simulink model "Karatsuba_Multiplier_64_Unsigned"  (R2012b)
settings: Solver=FixedStepDiscrete  SolverMode=SingleTasking  StartTime=0  StopTime=stopClock  RelTol=1e-3
libraries: xbsIndex_r4 x469
(part 2 of 3)

== system Karatsuba_Multiplier_64_Unsigned/AE_Multiplier_32_0/Barrel Shifter 9 ==
  Sel : Inport
  x : Inport  Port=2
  Mux : xbsIndex_r4/Mux  inputs=8  en=off  latency=0  precision=Full  arith_type=Unsigned  n_bits=17  bin_pt=0  quantization=Truncate  overflow=Wrap  dbl_ovrd=off  block_type=mux
  Shift1 : xbsIndex_r4/Shift  shift_dir=Left  shift_bits=1  en=off  latency=0  precision=User Defined  arith_type=Unsigned  n_bits=64  bin_pt=0  quantization=Truncate  overflow=Wrap  dbl_ovrd=off  block_type=shift
  Shift2 : xbsIndex_r4/Shift  shift_dir=Left  shift_bits=2  en=off  latency=0  precision=User Defined  arith_type=Unsigned  n_bits=64  bin_pt=0  quantization=Truncate  overflow=Wrap  dbl_ovrd=off  block_type=shift
  Shift3 : xbsIndex_r4/Shift  shift_dir=Left  shift_bits=3  en=off  latency=0  precision=User Defined  arith_type="Signed  (2's comp)"  n_bits=64  bin_pt=0  quantization=Truncate  overflow=Wrap  dbl_ovrd=off  block_type=shift
  Shift4 : xbsIndex_r4/Shift  shift_dir=Left  shift_bits=4  en=off  latency=0  precision=User Defined  arith_type=Unsigned  n_bits=64  bin_pt=0  quantization=Truncate  overflow=Wrap  dbl_ovrd=off  block_type=shift
  Shift5 : xbsIndex_r4/Shift  shift_dir=Left  shift_bits=5  en=off  latency=0  precision=User Defined  arith_type=Unsigned  n_bits=43  bin_pt=0  quantization=Truncate  overflow=Wrap  dbl_ovrd=off  block_type=shift
  Shift6 : xbsIndex_r4/Shift  shift_dir=Left  shift_bits=6  en=off  latency=0  precision=User Defined  arith_type=Unsigned  n_bits=64  bin_pt=0  quantization=Truncate  overflow=Wrap  dbl_ovrd=off  block_type=shift
  Shift7 : xbsIndex_r4/Shift  shift_dir=Left  shift_bits=7  en=off  latency=0  precision=User Defined  arith_type=Unsigned  n_bits=64  bin_pt=0  quantization=Truncate  overflow=Wrap  dbl_ovrd=off  block_type=shift
  y : Outport
  wires:
  Mux/1 -> y/1
  Sel/1 -> Mux/1
  x/1 -> Shift1/1, Shift2/1, Shift3/1, Shift4/1, Shift5/1, Shift6/1, Shift7/1, Mux/2
  Shift1/1 -> Mux/3
  Shift2/1 -> Mux/4
  Shift3/1 -> Mux/5
  Shift4/1 -> Mux/6
  Shift5/1 -> Mux/7
  Shift6/1 -> Mux/8
  Shift7/1 -> Mux/9

== system Karatsuba_Multiplier_64_Unsigned/AE_Multiplier_32_0/Encoder Slicer0 ==
  x : Inport
  Slice Enc a1 : xbsIndex_r4/Slice  nbits=3  boolean_output=off  mode=Lower Bit Location + Width  bit1=0  base1=MSB of Input  bit0=6  base0=LSB of Input  dbl_ovrd=off  block_type=slice
  Slice Enc a2 : xbsIndex_r4/Slice  nbits=3  boolean_output=off  mode=Lower Bit Location + Width  bit1=0  base1=MSB of Input  bit0=0  base0=LSB of Input  dbl_ovrd=off  block_type=slice
  Slice Enc s2 : xbsIndex_r4/Slice  nbits=1  boolean_output=on  mode=Lower Bit Location + Width  bit1=0  base1=MSB of Input  bit0=3  base0=LSB of Input  dbl_ovrd=off  block_type=slice
  Slice Enc t1 : xbsIndex_r4/Slice  nbits=2  boolean_output=off  mode=Upper Bit Location + Width  bit1=0  base1=MSB of Input  bit0=0  base0=MSB of Input  dbl_ovrd=off  block_type=slice
  Slice Enc t2 : xbsIndex_r4/Slice  nbits=2  boolean_output=off  mode=Lower Bit Location + Width  bit1=0  base1=MSB of Input  bit0=4  base0=LSB of Input  dbl_ovrd=off  block_type=slice
  t1 : Outport
  a1 : Outport  Port=2
  t2 : Outport  Port=3
  a2 : Outport  Port=4
  s2 : Outport  Port=5
  wires:
  Slice Enc t2/1 -> t2/1
  Slice Enc a1/1 -> a1/1
  Slice Enc a2/1 -> a2/1
  Slice Enc t1/1 -> t1/1
  Slice Enc s2/1 -> s2/1
  x/1 -> Slice Enc s2/1, Slice Enc a2/1, Slice Enc t1/1, Slice Enc a1/1, Slice Enc t2/1

== system Karatsuba_Multiplier_64_Unsigned/AE_Multiplier_32_0/Encoder Slicer1 ==
  x : Inport
  Slice Enc a1 : xbsIndex_r4/Slice  nbits=3  boolean_output=off  mode=Lower Bit Location + Width  bit1=0  base1=MSB of Input  bit0=6  base0=LSB of Input  dbl_ovrd=off  block_type=slice
  Slice Enc a2 : xbsIndex_r4/Slice  nbits=3  boolean_output=off  mode=Lower Bit Location + Width  bit1=0  base1=MSB of Input  bit0=0  base0=LSB of Input  dbl_ovrd=off  block_type=slice
  Slice Enc s2 : xbsIndex_r4/Slice  nbits=1  boolean_output=on  mode=Lower Bit Location + Width  bit1=0  base1=MSB of Input  bit0=3  base0=LSB of Input  dbl_ovrd=off  block_type=slice
  Slice Enc t1 : xbsIndex_r4/Slice  nbits=2  boolean_output=off  mode=Upper Bit Location + Width  bit1=0  base1=MSB of Input  bit0=0  base0=MSB of Input  dbl_ovrd=off  block_type=slice
  Slice Enc t2 : xbsIndex_r4/Slice  nbits=2  boolean_output=off  mode=Lower Bit Location + Width  bit1=0  base1=MSB of Input  bit0=4  base0=LSB of Input  dbl_ovrd=off  block_type=slice
  t1 : Outport
  a1 : Outport  Port=2
  t2 : Outport  Port=3
  a2 : Outport  Port=4
  s2 : Outport  Port=5
  wires:
  Slice Enc t2/1 -> t2/1
  Slice Enc a1/1 -> a1/1
  Slice Enc a2/1 -> a2/1
  Slice Enc t1/1 -> t1/1
  Slice Enc s2/1 -> s2/1
  x/1 -> Slice Enc s2/1, Slice Enc a2/1, Slice Enc t1/1, Slice Enc a1/1, Slice Enc t2/1

== system Karatsuba_Multiplier_64_Unsigned/AE_Multiplier_32_0/Encoder Slicer2 ==
  x : Inport
  Slice Enc a1 : xbsIndex_r4/Slice  nbits=3  boolean_output=off  mode=Lower Bit Location + Width  bit1=0  base1=MSB of Input  bit0=6  base0=LSB of Input  dbl_ovrd=off  block_type=slice
  Slice Enc a2 : xbsIndex_r4/Slice  nbits=3  boolean_output=off  mode=Lower Bit Location + Width  bit1=0  base1=MSB of Input  bit0=0  base0=LSB of Input  dbl_ovrd=off  block_type=slice
  Slice Enc s2 : xbsIndex_r4/Slice  nbits=1  boolean_output=on  mode=Lower Bit Location + Width  bit1=0  base1=MSB of Input  bit0=3  base0=LSB of Input  dbl_ovrd=off  block_type=slice
  Slice Enc t1 : xbsIndex_r4/Slice  nbits=2  boolean_output=off  mode=Upper Bit Location + Width  bit1=0  base1=MSB of Input  bit0=0  base0=MSB of Input  dbl_ovrd=off  block_type=slice
  Slice Enc t2 : xbsIndex_r4/Slice  nbits=2  boolean_output=off  mode=Lower Bit Location + Width  bit1=0  base1=MSB of Input  bit0=4  base0=LSB of Input  dbl_ovrd=off  block_type=slice
  t1 : Outport
  a1 : Outport  Port=2
  t2 : Outport  Port=3
  a2 : Outport  Port=4
  s2 : Outport  Port=5
  wires:
  Slice Enc t2/1 -> t2/1
  Slice Enc a1/1 -> a1/1
  Slice Enc a2/1 -> a2/1
  Slice Enc t1/1 -> t1/1
  Slice Enc s2/1 -> s2/1
  x/1 -> Slice Enc s2/1, Slice Enc a2/1, Slice Enc t1/1, Slice Enc a1/1, Slice Enc t2/1

== system Karatsuba_Multiplier_64_Unsigned/AE_Multiplier_32_0/Encoder Slicer3 ==
  x : Inport
  Slice Enc a1 : xbsIndex_r4/Slice  nbits=3  boolean_output=off  mode=Lower Bit Location + Width  bit1=0  base1=MSB of Input  bit0=6  base0=LSB of Input  dbl_ovrd=off  block_type=slice
  Slice Enc a2 : xbsIndex_r4/Slice  nbits=3  boolean_output=off  mode=Lower Bit Location + Width  bit1=0  base1=MSB of Input  bit0=0  base0=LSB of Input  dbl_ovrd=off  block_type=slice
  Slice Enc s2 : xbsIndex_r4/Slice  nbits=1  boolean_output=on  mode=Lower Bit Location + Width  bit1=0  base1=MSB of Input  bit0=3  base0=LSB of Input  dbl_ovrd=off  block_type=slice
  Slice Enc t1 : xbsIndex_r4/Slice  nbits=2  boolean_output=off  mode=Upper Bit Location + Width  bit1=0  base1=MSB of Input  bit0=0  base0=MSB of Input  dbl_ovrd=off  block_type=slice
  Slice Enc t2 : xbsIndex_r4/Slice  nbits=2  boolean_output=off  mode=Lower Bit Location + Width  bit1=0  base1=MSB of Input  bit0=4  base0=LSB of Input  dbl_ovrd=off  block_type=slice
  t1 : Outport
  a1 : Outport  Port=2
  t2 : Outport  Port=3
  a2 : Outport  Port=4
  s2 : Outport  Port=5
  wires:
  Slice Enc t2/1 -> t2/1
  Slice Enc a1/1 -> a1/1
  Slice Enc a2/1 -> a2/1
  Slice Enc t1/1 -> t1/1
  Slice Enc s2/1 -> s2/1
  x/1 -> Slice Enc s2/1, Slice Enc a2/1, Slice Enc t1/1, Slice Enc a1/1, Slice Enc t2/1

== system Karatsuba_Multiplier_64_Unsigned/AE_Multiplier_32_0/Encoder Slicer4 ==
  x : Inport
  Slice Enc a1 : xbsIndex_r4/Slice  nbits=3  boolean_output=off  mode=Lower Bit Location + Width  bit1=0  base1=MSB of Input  bit0=6  base0=LSB of Input  dbl_ovrd=off  block_type=slice
  Slice Enc a2 : xbsIndex_r4/Slice  nbits=3  boolean_output=off  mode=Lower Bit Location + Width  bit1=0  base1=MSB of Input  bit0=0  base0=LSB of Input  dbl_ovrd=off  block_type=slice
  Slice Enc s2 : xbsIndex_r4/Slice  nbits=1  boolean_output=on  mode=Lower Bit Location + Width  bit1=0  base1=MSB of Input  bit0=3  base0=LSB of Input  dbl_ovrd=off  block_type=slice
  Slice Enc t1 : xbsIndex_r4/Slice  nbits=2  boolean_output=off  mode=Upper Bit Location + Width  bit1=0  base1=MSB of Input  bit0=0  base0=MSB of Input  dbl_ovrd=off  block_type=slice
  Slice Enc t2 : xbsIndex_r4/Slice  nbits=2  boolean_output=off  mode=Lower Bit Location + Width  bit1=0  base1=MSB of Input  bit0=4  base0=LSB of Input  dbl_ovrd=off  block_type=slice
  t1 : Outport
  a1 : Outport  Port=2
  t2 : Outport  Port=3
  a2 : Outport  Port=4
  s2 : Outport  Port=5
  wires:
  Slice Enc t2/1 -> t2/1
  Slice Enc a1/1 -> a1/1
  Slice Enc a2/1 -> a2/1
  Slice Enc t1/1 -> t1/1
  Slice Enc s2/1 -> s2/1
  x/1 -> Slice Enc s2/1, Slice Enc a2/1, Slice Enc t1/1, Slice Enc a1/1, Slice Enc t2/1

== system Karatsuba_Multiplier_64_Unsigned/AE_Multiplier_32_1/3B Multiplier ==
  x : Inport
  AddSub : xbsIndex_r4/AddSub  mode=Addition  use_carryin=off  use_carryout=off  en=off  latency=0  precision=User Defined  arith_type=Unsigned  n_bits=64  bin_pt=0  quantization=Truncate  overflow=Wrap  dbl_ovrd=off  use_behavioral_HDL=off  hw_selection=Fabric  pipelined=on  block_type=addsub
  Shift : xbsIndex_r4/Shift  shift_dir=Left  shift_bits=1  en=off  latency=0  precision=User Defined  arith_type=Unsigned  n_bits=64  bin_pt=0  quantization=Truncate  overflow=Wrap  dbl_ovrd=off  block_type=shift
  y : Outport
  wires:
  x/1 -> Shift/1, AddSub/2
  AddSub/1 -> y/1
  Shift/1 -> AddSub/1

== system Karatsuba_Multiplier_64_Unsigned/AE_Multiplier_32_1/5B Multiplier ==
  x : Inport
  AddSub1 : xbsIndex_r4/AddSub  mode=Addition  use_carryin=off  use_carryout=off  en=off  latency=0  precision=User Defined  arith_type=Unsigned  n_bits=64  bin_pt=0  quantization=Truncate  overflow=Wrap  dbl_ovrd=off  use_behavioral_HDL=off  hw_selection=Fabric  pipelined=on  block_type=addsub
  Shift1 : xbsIndex_r4/Shift  shift_dir=Left  shift_bits=2  en=off  latency=0  precision=User Defined  arith_type=Unsigned  n_bits=64  bin_pt=0  quantization=Truncate  overflow=Wrap  dbl_ovrd=off  block_type=shift
  y : Outport
  wires:
  x/1 -> AddSub1/2, Shift1/1
  Shift1/1 -> AddSub1/1
  AddSub1/1 -> y/1

== system Karatsuba_Multiplier_64_Unsigned/AE_Multiplier_32_1/7B Multiplier ==
  x : Inport
  AddSub2 : xbsIndex_r4/AddSub  mode=Subtraction  use_carryin=off  use_carryout=off  en=off  latency=0  precision=User Defined  arith_type=Unsigned  n_bits=64  bin_pt=0  quantization=Truncate  overflow=Wrap  dbl_ovrd=off  use_behavioral_HDL=off  hw_selection=Fabric  pipelined=on  block_type=addsub
  Shift2 : xbsIndex_r4/Shift  shift_dir=Left  shift_bits=3  en=off  latency=0  precision=User Defined  arith_type=Unsigned  n_bits=64  bin_pt=0  quantization=Truncate  overflow=Wrap  dbl_ovrd=off  block_type=shift
  y : Outport
  wires:
  AddSub2/1 -> y/1
  Shift2/1 -> AddSub2/1
  x/1 -> Shift2/1, AddSub2/2

== system Karatsuba_Multiplier_64_Unsigned/AE_Multiplier_32_1/Barrel Shifter 0 ==
  Sel : Inport
  x : Inport  Port=2
  Mux : xbsIndex_r4/Mux  inputs=8  en=off  latency=0  precision=Full  arith_type=Unsigned  n_bits=17  bin_pt=0  quantization=Truncate  overflow=Wrap  dbl_ovrd=off  block_type=mux
  Shift1 : xbsIndex_r4/Shift  shift_dir=Left  shift_bits=1  en=off  latency=0  precision=User Defined  arith_type=Unsigned  n_bits=64  bin_pt=0  quantization=Truncate  overflow=Wrap  dbl_ovrd=off  block_type=shift
  Shift2 : xbsIndex_r4/Shift  shift_dir=Left  shift_bits=2  en=off  latency=0  precision=User Defined  arith_type=Unsigned  n_bits=64  bin_pt=0  quantization=Truncate  overflow=Wrap  dbl_ovrd=off  block_type=shift
  Shift3 : xbsIndex_r4/Shift  shift_dir=Left  shift_bits=3  en=off  latency=0  precision=User Defined  arith_type="Signed  (2's comp)"  n_bits=64  bin_pt=0  quantization=Truncate  overflow=Wrap  dbl_ovrd=off  block_type=shift
  Shift4 : xbsIndex_r4/Shift  shift_dir=Left  shift_bits=4  en=off  latency=0  precision=User Defined  arith_type=Unsigned  n_bits=64  bin_pt=0  quantization=Truncate  overflow=Wrap  dbl_ovrd=off  block_type=shift
  Shift5 : xbsIndex_r4/Shift  shift_dir=Left  shift_bits=5  en=off  latency=0  precision=User Defined  arith_type=Unsigned  n_bits=43  bin_pt=0  quantization=Truncate  overflow=Wrap  dbl_ovrd=off  block_type=shift
  Shift6 : xbsIndex_r4/Shift  shift_dir=Left  shift_bits=6  en=off  latency=0  precision=User Defined  arith_type=Unsigned  n_bits=64  bin_pt=0  quantization=Truncate  overflow=Wrap  dbl_ovrd=off  block_type=shift
  Shift7 : xbsIndex_r4/Shift  shift_dir=Left  shift_bits=7  en=off  latency=0  precision=User Defined  arith_type=Unsigned  n_bits=64  bin_pt=0  quantization=Truncate  overflow=Wrap  dbl_ovrd=off  block_type=shift
  y : Outport
  wires:
  Mux/1 -> y/1
  Sel/1 -> Mux/1
  x/1 -> Shift1/1, Shift2/1, Shift3/1, Shift4/1, Shift5/1, Shift6/1, Shift7/1, Mux/2
  Shift1/1 -> Mux/3
  Shift2/1 -> Mux/4
  Shift3/1 -> Mux/5
  Shift4/1 -> Mux/6
  Shift5/1 -> Mux/7
  Shift6/1 -> Mux/8
  Shift7/1 -> Mux/9

== system Karatsuba_Multiplier_64_Unsigned/AE_Multiplier_32_1/Barrel Shifter 1 ==
  Sel : Inport
  x : Inport  Port=2
  Mux : xbsIndex_r4/Mux  inputs=8  en=off  latency=0  precision=Full  arith_type=Unsigned  n_bits=17  bin_pt=0  quantization=Truncate  overflow=Wrap  dbl_ovrd=off  block_type=mux
  Shift1 : xbsIndex_r4/Shift  shift_dir=Left  shift_bits=1  en=off  latency=0  precision=User Defined  arith_type=Unsigned  n_bits=64  bin_pt=0  quantization=Truncate  overflow=Wrap  dbl_ovrd=off  block_type=shift
  Shift2 : xbsIndex_r4/Shift  shift_dir=Left  shift_bits=2  en=off  latency=0  precision=User Defined  arith_type=Unsigned  n_bits=64  bin_pt=0  quantization=Truncate  overflow=Wrap  dbl_ovrd=off  block_type=shift
  Shift3 : xbsIndex_r4/Shift  shift_dir=Left  shift_bits=3  en=off  latency=0  precision=User Defined  arith_type="Signed  (2's comp)"  n_bits=64  bin_pt=0  quantization=Truncate  overflow=Wrap  dbl_ovrd=off  block_type=shift
  Shift4 : xbsIndex_r4/Shift  shift_dir=Left  shift_bits=4  en=off  latency=0  precision=User Defined  arith_type=Unsigned  n_bits=64  bin_pt=0  quantization=Truncate  overflow=Wrap  dbl_ovrd=off  block_type=shift
  Shift5 : xbsIndex_r4/Shift  shift_dir=Left  shift_bits=5  en=off  latency=0  precision=User Defined  arith_type=Unsigned  n_bits=43  bin_pt=0  quantization=Truncate  overflow=Wrap  dbl_ovrd=off  block_type=shift
  Shift6 : xbsIndex_r4/Shift  shift_dir=Left  shift_bits=6  en=off  latency=0  precision=User Defined  arith_type=Unsigned  n_bits=64  bin_pt=0  quantization=Truncate  overflow=Wrap  dbl_ovrd=off  block_type=shift
  Shift7 : xbsIndex_r4/Shift  shift_dir=Left  shift_bits=7  en=off  latency=0  precision=User Defined  arith_type=Unsigned  n_bits=64  bin_pt=0  quantization=Truncate  overflow=Wrap  dbl_ovrd=off  block_type=shift
  y : Outport
  wires:
  Mux/1 -> y/1
  Sel/1 -> Mux/1
  x/1 -> Shift1/1, Shift2/1, Shift3/1, Shift4/1, Shift5/1, Shift6/1, Shift7/1, Mux/2
  Shift1/1 -> Mux/3
  Shift2/1 -> Mux/4
  Shift3/1 -> Mux/5
  Shift4/1 -> Mux/6
  Shift5/1 -> Mux/7
  Shift6/1 -> Mux/8
  Shift7/1 -> Mux/9

== system Karatsuba_Multiplier_64_Unsigned/AE_Multiplier_32_1/Barrel Shifter 2 ==
  Sel : Inport
  x : Inport  Port=2
  Mux : xbsIndex_r4/Mux  inputs=8  en=off  latency=0  precision=Full  arith_type=Unsigned  n_bits=17  bin_pt=0  quantization=Truncate  overflow=Wrap  dbl_ovrd=off  block_type=mux
  Shift1 : xbsIndex_r4/Shift  shift_dir=Left  shift_bits=1  en=off  latency=0  precision=User Defined  arith_type=Unsigned  n_bits=64  bin_pt=0  quantization=Truncate  overflow=Wrap  dbl_ovrd=off  block_type=shift
  Shift2 : xbsIndex_r4/Shift  shift_dir=Left  shift_bits=2  en=off  latency=0  precision=User Defined  arith_type=Unsigned  n_bits=64  bin_pt=0  quantization=Truncate  overflow=Wrap  dbl_ovrd=off  block_type=shift
  Shift3 : xbsIndex_r4/Shift  shift_dir=Left  shift_bits=3  en=off  latency=0  precision=User Defined  arith_type="Signed  (2's comp)"  n_bits=64  bin_pt=0  quantization=Truncate  overflow=Wrap  dbl_ovrd=off  block_type=shift
  Shift4 : xbsIndex_r4/Shift  shift_dir=Left  shift_bits=4  en=off  latency=0  precision=User Defined  arith_type=Unsigned  n_bits=64  bin_pt=0  quantization=Truncate  overflow=Wrap  dbl_ovrd=off  block_type=shift
  Shift5 : xbsIndex_r4/Shift  shift_dir=Left  shift_bits=5  en=off  latency=0  precision=User Defined  arith_type=Unsigned  n_bits=43  bin_pt=0  quantization=Truncate  overflow=Wrap  dbl_ovrd=off  block_type=shift
  Shift6 : xbsIndex_r4/Shift  shift_dir=Left  shift_bits=6  en=off  latency=0  precision=User Defined  arith_type=Unsigned  n_bits=64  bin_pt=0  quantization=Truncate  overflow=Wrap  dbl_ovrd=off  block_type=shift
  Shift7 : xbsIndex_r4/Shift  shift_dir=Left  shift_bits=7  en=off  latency=0  precision=User Defined  arith_type=Unsigned  n_bits=64  bin_pt=0  quantization=Truncate  overflow=Wrap  dbl_ovrd=off  block_type=shift
  y : Outport
  wires:
  Mux/1 -> y/1
  Sel/1 -> Mux/1
  x/1 -> Shift1/1, Shift2/1, Shift3/1, Shift4/1, Shift5/1, Shift6/1, Shift7/1, Mux/2
  Shift1/1 -> Mux/3
  Shift2/1 -> Mux/4
  Shift3/1 -> Mux/5
  Shift4/1 -> Mux/6
  Shift5/1 -> Mux/7
  Shift6/1 -> Mux/8
  Shift7/1 -> Mux/9

== system Karatsuba_Multiplier_64_Unsigned/AE_Multiplier_32_1/Barrel Shifter 3 ==
  Sel : Inport
  x : Inport  Port=2
  Mux : xbsIndex_r4/Mux  inputs=8  en=off  latency=0  precision=Full  arith_type=Unsigned  n_bits=17  bin_pt=0  quantization=Truncate  overflow=Wrap  dbl_ovrd=off  block_type=mux
  Shift1 : xbsIndex_r4/Shift  shift_dir=Left  shift_bits=1  en=off  latency=0  precision=User Defined  arith_type=Unsigned  n_bits=64  bin_pt=0  quantization=Truncate  overflow=Wrap  dbl_ovrd=off  block_type=shift
  Shift2 : xbsIndex_r4/Shift  shift_dir=Left  shift_bits=2  en=off  latency=0  precision=User Defined  arith_type=Unsigned  n_bits=64  bin_pt=0  quantization=Truncate  overflow=Wrap  dbl_ovrd=off  block_type=shift
  Shift3 : xbsIndex_r4/Shift  shift_dir=Left  shift_bits=3  en=off  latency=0  precision=User Defined  arith_type="Signed  (2's comp)"  n_bits=64  bin_pt=0  quantization=Truncate  overflow=Wrap  dbl_ovrd=off  block_type=shift
  Shift4 : xbsIndex_r4/Shift  shift_dir=Left  shift_bits=4  en=off  latency=0  precision=User Defined  arith_type=Unsigned  n_bits=64  bin_pt=0  quantization=Truncate  overflow=Wrap  dbl_ovrd=off  block_type=shift
  Shift5 : xbsIndex_r4/Shift  shift_dir=Left  shift_bits=5  en=off  latency=0  precision=User Defined  arith_type=Unsigned  n_bits=43  bin_pt=0  quantization=Truncate  overflow=Wrap  dbl_ovrd=off  block_type=shift
  Shift6 : xbsIndex_r4/Shift  shift_dir=Left  shift_bits=6  en=off  latency=0  precision=User Defined  arith_type=Unsigned  n_bits=64  bin_pt=0  quantization=Truncate  overflow=Wrap  dbl_ovrd=off  block_type=shift
  Shift7 : xbsIndex_r4/Shift  shift_dir=Left  shift_bits=7  en=off  latency=0  precision=User Defined  arith_type=Unsigned  n_bits=64  bin_pt=0  quantization=Truncate  overflow=Wrap  dbl_ovrd=off  block_type=shift
  y : Outport
  wires:
  Mux/1 -> y/1
  Sel/1 -> Mux/1
  x/1 -> Shift1/1, Shift2/1, Shift3/1, Shift4/1, Shift5/1, Shift6/1, Shift7/1, Mux/2
  Shift1/1 -> Mux/3
  Shift2/1 -> Mux/4
  Shift3/1 -> Mux/5
  Shift4/1 -> Mux/6
  Shift5/1 -> Mux/7
  Shift6/1 -> Mux/8
  Shift7/1 -> Mux/9

== system Karatsuba_Multiplier_64_Unsigned/AE_Multiplier_32_1/Barrel Shifter 4 ==
  Sel : Inport
  x : Inport  Port=2
  Mux : xbsIndex_r4/Mux  inputs=8  en=off  latency=0  precision=Full  arith_type=Unsigned  n_bits=17  bin_pt=0  quantization=Truncate  overflow=Wrap  dbl_ovrd=off  block_type=mux
  Shift1 : xbsIndex_r4/Shift  shift_dir=Left  shift_bits=1  en=off  latency=0  precision=User Defined  arith_type=Unsigned  n_bits=64  bin_pt=0  quantization=Truncate  overflow=Wrap  dbl_ovrd=off  block_type=shift
  Shift2 : xbsIndex_r4/Shift  shift_dir=Left  shift_bits=2  en=off  latency=0  precision=User Defined  arith_type=Unsigned  n_bits=64  bin_pt=0  quantization=Truncate  overflow=Wrap  dbl_ovrd=off  block_type=shift
  Shift3 : xbsIndex_r4/Shift  shift_dir=Left  shift_bits=3  en=off  latency=0  precision=User Defined  arith_type="Signed  (2's comp)"  n_bits=64  bin_pt=0  quantization=Truncate  overflow=Wrap  dbl_ovrd=off  block_type=shift
  Shift4 : xbsIndex_r4/Shift  shift_dir=Left  shift_bits=4  en=off  latency=0  precision=User Defined  arith_type=Unsigned  n_bits=64  bin_pt=0  quantization=Truncate  overflow=Wrap  dbl_ovrd=off  block_type=shift
  Shift5 : xbsIndex_r4/Shift  shift_dir=Left  shift_bits=5  en=off  latency=0  precision=User Defined  arith_type=Unsigned  n_bits=43  bin_pt=0  quantization=Truncate  overflow=Wrap  dbl_ovrd=off  block_type=shift
  Shift6 : xbsIndex_r4/Shift  shift_dir=Left  shift_bits=6  en=off  latency=0  precision=User Defined  arith_type=Unsigned  n_bits=64  bin_pt=0  quantization=Truncate  overflow=Wrap  dbl_ovrd=off  block_type=shift
  Shift7 : xbsIndex_r4/Shift  shift_dir=Left  shift_bits=7  en=off  latency=0  precision=User Defined  arith_type=Unsigned  n_bits=64  bin_pt=0  quantization=Truncate  overflow=Wrap  dbl_ovrd=off  block_type=shift
  y : Outport
  wires:
  Mux/1 -> y/1
  Sel/1 -> Mux/1
  x/1 -> Shift1/1, Shift2/1, Shift3/1, Shift4/1, Shift5/1, Shift6/1, Shift7/1, Mux/2
  Shift1/1 -> Mux/3
  Shift2/1 -> Mux/4
  Shift3/1 -> Mux/5
  Shift4/1 -> Mux/6
  Shift5/1 -> Mux/7
  Shift6/1 -> Mux/8
  Shift7/1 -> Mux/9

== system Karatsuba_Multiplier_64_Unsigned/AE_Multiplier_32_1/Barrel Shifter 5 ==
  Sel : Inport
  x : Inport  Port=2
  Mux : xbsIndex_r4/Mux  inputs=8  en=off  latency=0  precision=Full  arith_type=Unsigned  n_bits=17  bin_pt=0  quantization=Truncate  overflow=Wrap  dbl_ovrd=off  block_type=mux
  Shift1 : xbsIndex_r4/Shift  shift_dir=Left  shift_bits=1  en=off  latency=0  precision=User Defined  arith_type=Unsigned  n_bits=64  bin_pt=0  quantization=Truncate  overflow=Wrap  dbl_ovrd=off  block_type=shift
  Shift2 : xbsIndex_r4/Shift  shift_dir=Left  shift_bits=2  en=off  latency=0  precision=User Defined  arith_type=Unsigned  n_bits=64  bin_pt=0  quantization=Truncate  overflow=Wrap  dbl_ovrd=off  block_type=shift
  Shift3 : xbsIndex_r4/Shift  shift_dir=Left  shift_bits=3  en=off  latency=0  precision=User Defined  arith_type="Signed  (2's comp)"  n_bits=64  bin_pt=0  quantization=Truncate  overflow=Wrap  dbl_ovrd=off  block_type=shift
  Shift4 : xbsIndex_r4/Shift  shift_dir=Left  shift_bits=4  en=off  latency=0  precision=User Defined  arith_type=Unsigned  n_bits=64  bin_pt=0  quantization=Truncate  overflow=Wrap  dbl_ovrd=off  block_type=shift
  Shift5 : xbsIndex_r4/Shift  shift_dir=Left  shift_bits=5  en=off  latency=0  precision=User Defined  arith_type=Unsigned  n_bits=43  bin_pt=0  quantization=Truncate  overflow=Wrap  dbl_ovrd=off  block_type=shift
  Shift6 : xbsIndex_r4/Shift  shift_dir=Left  shift_bits=6  en=off  latency=0  precision=User Defined  arith_type=Unsigned  n_bits=64  bin_pt=0  quantization=Truncate  overflow=Wrap  dbl_ovrd=off  block_type=shift
  Shift7 : xbsIndex_r4/Shift  shift_dir=Left  shift_bits=7  en=off  latency=0  precision=User Defined  arith_type=Unsigned  n_bits=64  bin_pt=0  quantization=Truncate  overflow=Wrap  dbl_ovrd=off  block_type=shift
  y : Outport
  wires:
  Mux/1 -> y/1
  Sel/1 -> Mux/1
  x/1 -> Shift1/1, Shift2/1, Shift3/1, Shift4/1, Shift5/1, Shift6/1, Shift7/1, Mux/2
  Shift1/1 -> Mux/3
  Shift2/1 -> Mux/4
  Shift3/1 -> Mux/5
  Shift4/1 -> Mux/6
  Shift5/1 -> Mux/7
  Shift6/1 -> Mux/8
  Shift7/1 -> Mux/9

== system Karatsuba_Multiplier_64_Unsigned/AE_Multiplier_32_1/Barrel Shifter 6 ==
  Sel : Inport
  x : Inport  Port=2
  Mux : xbsIndex_r4/Mux  inputs=8  en=off  latency=0  precision=Full  arith_type=Unsigned  n_bits=17  bin_pt=0  quantization=Truncate  overflow=Wrap  dbl_ovrd=off  block_type=mux
  Shift1 : xbsIndex_r4/Shift  shift_dir=Left  shift_bits=1  en=off  latency=0  precision=User Defined  arith_type=Unsigned  n_bits=64  bin_pt=0  quantization=Truncate  overflow=Wrap  dbl_ovrd=off  block_type=shift
  Shift2 : xbsIndex_r4/Shift  shift_dir=Left  shift_bits=2  en=off  latency=0  precision=User Defined  arith_type=Unsigned  n_bits=64  bin_pt=0  quantization=Truncate  overflow=Wrap  dbl_ovrd=off  block_type=shift
  Shift3 : xbsIndex_r4/Shift  shift_dir=Left  shift_bits=3  en=off  latency=0  precision=User Defined  arith_type="Signed  (2's comp)"  n_bits=64  bin_pt=0  quantization=Truncate  overflow=Wrap  dbl_ovrd=off  block_type=shift
  Shift4 : xbsIndex_r4/Shift  shift_dir=Left  shift_bits=4  en=off  latency=0  precision=User Defined  arith_type=Unsigned  n_bits=64  bin_pt=0  quantization=Truncate  overflow=Wrap  dbl_ovrd=off  block_type=shift
  Shift5 : xbsIndex_r4/Shift  shift_dir=Left  shift_bits=5  en=off  latency=0  precision=User Defined  arith_type=Unsigned  n_bits=43  bin_pt=0  quantization=Truncate  overflow=Wrap  dbl_ovrd=off  block_type=shift
  Shift6 : xbsIndex_r4/Shift  shift_dir=Left  shift_bits=6  en=off  latency=0  precision=User Defined  arith_type=Unsigned  n_bits=64  bin_pt=0  quantization=Truncate  overflow=Wrap  dbl_ovrd=off  block_type=shift
  Shift7 : xbsIndex_r4/Shift  shift_dir=Left  shift_bits=7  en=off  latency=0  precision=User Defined  arith_type=Unsigned  n_bits=64  bin_pt=0  quantization=Truncate  overflow=Wrap  dbl_ovrd=off  block_type=shift
  y : Outport
  wires:
  Mux/1 -> y/1
  Sel/1 -> Mux/1
  x/1 -> Shift1/1, Shift2/1, Shift3/1, Shift4/1, Shift5/1, Shift6/1, Shift7/1, Mux/2
  Shift1/1 -> Mux/3
  Shift2/1 -> Mux/4
  Shift3/1 -> Mux/5
  Shift4/1 -> Mux/6
  Shift5/1 -> Mux/7
  Shift6/1 -> Mux/8
  Shift7/1 -> Mux/9

== system Karatsuba_Multiplier_64_Unsigned/AE_Multiplier_32_1/Barrel Shifter 7 ==
  Sel : Inport
  x : Inport  Port=2
  Mux : xbsIndex_r4/Mux  inputs=8  en=off  latency=0  precision=Full  arith_type=Unsigned  n_bits=17  bin_pt=0  quantization=Truncate  overflow=Wrap  dbl_ovrd=off  block_type=mux
  Shift1 : xbsIndex_r4/Shift  shift_dir=Left  shift_bits=1  en=off  latency=0  precision=User Defined  arith_type=Unsigned  n_bits=64  bin_pt=0  quantization=Truncate  overflow=Wrap  dbl_ovrd=off  block_type=shift
  Shift2 : xbsIndex_r4/Shift  shift_dir=Left  shift_bits=2  en=off  latency=0  precision=User Defined  arith_type=Unsigned  n_bits=64  bin_pt=0  quantization=Truncate  overflow=Wrap  dbl_ovrd=off  block_type=shift
  Shift3 : xbsIndex_r4/Shift  shift_dir=Left  shift_bits=3  en=off  latency=0  precision=User Defined  arith_type="Signed  (2's comp)"  n_bits=64  bin_pt=0  quantization=Truncate  overflow=Wrap  dbl_ovrd=off  block_type=shift
  Shift4 : xbsIndex_r4/Shift  shift_dir=Left  shift_bits=4  en=off  latency=0  precision=User Defined  arith_type=Unsigned  n_bits=64  bin_pt=0  quantization=Truncate  overflow=Wrap  dbl_ovrd=off  block_type=shift
  Shift5 : xbsIndex_r4/Shift  shift_dir=Left  shift_bits=5  en=off  latency=0  precision=User Defined  arith_type=Unsigned  n_bits=43  bin_pt=0  quantization=Truncate  overflow=Wrap  dbl_ovrd=off  block_type=shift
  Shift6 : xbsIndex_r4/Shift  shift_dir=Left  shift_bits=6  en=off  latency=0  precision=User Defined  arith_type=Unsigned  n_bits=64  bin_pt=0  quantization=Truncate  overflow=Wrap  dbl_ovrd=off  block_type=shift
  Shift7 : xbsIndex_r4/Shift  shift_dir=Left  shift_bits=7  en=off  latency=0  precision=User Defined  arith_type=Unsigned  n_bits=64  bin_pt=0  quantization=Truncate  overflow=Wrap  dbl_ovrd=off  block_type=shift
  y : Outport
  wires:
  Mux/1 -> y/1
  Sel/1 -> Mux/1
  x/1 -> Shift1/1, Shift2/1, Shift3/1, Shift4/1, Shift5/1, Shift6/1, Shift7/1, Mux/2
  Shift1/1 -> Mux/3
  Shift2/1 -> Mux/4
  Shift3/1 -> Mux/5
  Shift4/1 -> Mux/6
  Shift5/1 -> Mux/7
  Shift6/1 -> Mux/8
  Shift7/1 -> Mux/9

== system Karatsuba_Multiplier_64_Unsigned/AE_Multiplier_32_1/Barrel Shifter 8 ==
  Sel : Inport
  x : Inport  Port=2
  Mux : xbsIndex_r4/Mux  inputs=8  en=off  latency=0  precision=Full  arith_type=Unsigned  n_bits=17  bin_pt=0  quantization=Truncate  overflow=Wrap  dbl_ovrd=off  block_type=mux
  Shift1 : xbsIndex_r4/Shift  shift_dir=Left  shift_bits=1  en=off  latency=0  precision=User Defined  arith_type=Unsigned  n_bits=64  bin_pt=0  quantization=Truncate  overflow=Wrap  dbl_ovrd=off  block_type=shift
  Shift2 : xbsIndex_r4/Shift  shift_dir=Left  shift_bits=2  en=off  latency=0  precision=User Defined  arith_type=Unsigned  n_bits=64  bin_pt=0  quantization=Truncate  overflow=Wrap  dbl_ovrd=off  block_type=shift
  Shift3 : xbsIndex_r4/Shift  shift_dir=Left  shift_bits=3  en=off  latency=0  precision=User Defined  arith_type="Signed  (2's comp)"  n_bits=64  bin_pt=0  quantization=Truncate  overflow=Wrap  dbl_ovrd=off  block_type=shift
  Shift4 : xbsIndex_r4/Shift  shift_dir=Left  shift_bits=4  en=off  latency=0  precision=User Defined  arith_type=Unsigned  n_bits=64  bin_pt=0  quantization=Truncate  overflow=Wrap  dbl_ovrd=off  block_type=shift
  Shift5 : xbsIndex_r4/Shift  shift_dir=Left  shift_bits=5  en=off  latency=0  precision=User Defined  arith_type=Unsigned  n_bits=43  bin_pt=0  quantization=Truncate  overflow=Wrap  dbl_ovrd=off  block_type=shift
  Shift6 : xbsIndex_r4/Shift  shift_dir=Left  shift_bits=6  en=off  latency=0  precision=User Defined  arith_type=Unsigned  n_bits=64  bin_pt=0  quantization=Truncate  overflow=Wrap  dbl_ovrd=off  block_type=shift
  Shift7 : xbsIndex_r4/Shift  shift_dir=Left  shift_bits=7  en=off  latency=0  precision=User Defined  arith_type=Unsigned  n_bits=64  bin_pt=0  quantization=Truncate  overflow=Wrap  dbl_ovrd=off  block_type=shift
  y : Outport
  wires:
  Mux/1 -> y/1
  Sel/1 -> Mux/1
  x/1 -> Shift1/1, Shift2/1, Shift3/1, Shift4/1, Shift5/1, Shift6/1, Shift7/1, Mux/2
  Shift1/1 -> Mux/3
  Shift2/1 -> Mux/4
  Shift3/1 -> Mux/5
  Shift4/1 -> Mux/6
  Shift5/1 -> Mux/7
  Shift6/1 -> Mux/8
  Shift7/1 -> Mux/9

== system Karatsuba_Multiplier_64_Unsigned/AE_Multiplier_32_1/Barrel Shifter 9 ==
  Sel : Inport
  x : Inport  Port=2
  Mux : xbsIndex_r4/Mux  inputs=8  en=off  latency=0  precision=Full  arith_type=Unsigned  n_bits=17  bin_pt=0  quantization=Truncate  overflow=Wrap  dbl_ovrd=off  block_type=mux
  Shift1 : xbsIndex_r4/Shift  shift_dir=Left  shift_bits=1  en=off  latency=0  precision=User Defined  arith_type=Unsigned  n_bits=64  bin_pt=0  quantization=Truncate  overflow=Wrap  dbl_ovrd=off  block_type=shift
  Shift2 : xbsIndex_r4/Shift  shift_dir=Left  shift_bits=2  en=off  latency=0  precision=User Defined  arith_type=Unsigned  n_bits=64  bin_pt=0  quantization=Truncate  overflow=Wrap  dbl_ovrd=off  block_type=shift
  Shift3 : xbsIndex_r4/Shift  shift_dir=Left  shift_bits=3  en=off  latency=0  precision=User Defined  arith_type="Signed  (2's comp)"  n_bits=64  bin_pt=0  quantization=Truncate  overflow=Wrap  dbl_ovrd=off  block_type=shift
  Shift4 : xbsIndex_r4/Shift  shift_dir=Left  shift_bits=4  en=off  latency=0  precision=User Defined  arith_type=Unsigned  n_bits=64  bin_pt=0  quantization=Truncate  overflow=Wrap  dbl_ovrd=off  block_type=shift
  Shift5 : xbsIndex_r4/Shift  shift_dir=Left  shift_bits=5  en=off  latency=0  precision=User Defined  arith_type=Unsigned  n_bits=43  bin_pt=0  quantization=Truncate  overflow=Wrap  dbl_ovrd=off  block_type=shift
  Shift6 : xbsIndex_r4/Shift  shift_dir=Left  shift_bits=6  en=off  latency=0  precision=User Defined  arith_type=Unsigned  n_bits=64  bin_pt=0  quantization=Truncate  overflow=Wrap  dbl_ovrd=off  block_type=shift
  Shift7 : xbsIndex_r4/Shift  shift_dir=Left  shift_bits=7  en=off  latency=0  precision=User Defined  arith_type=Unsigned  n_bits=64  bin_pt=0  quantization=Truncate  overflow=Wrap  dbl_ovrd=off  block_type=shift
  y : Outport
  wires:
  Mux/1 -> y/1
  Sel/1 -> Mux/1
  x/1 -> Shift1/1, Shift2/1, Shift3/1, Shift4/1, Shift5/1, Shift6/1, Shift7/1, Mux/2
  Shift1/1 -> Mux/3
  Shift2/1 -> Mux/4
  Shift3/1 -> Mux/5
  Shift4/1 -> Mux/6
  Shift5/1 -> Mux/7
  Shift6/1 -> Mux/8
  Shift7/1 -> Mux/9

== system Karatsuba_Multiplier_64_Unsigned/AE_Multiplier_32_1/Encoder Slicer0 ==
  x : Inport
  Slice Enc a1 : xbsIndex_r4/Slice  nbits=3  boolean_output=off  mode=Lower Bit Location + Width  bit1=0  base1=MSB of Input  bit0=6  base0=LSB of Input  dbl_ovrd=off  block_type=slice
  Slice Enc a2 : xbsIndex_r4/Slice  nbits=3  boolean_output=off  mode=Lower Bit Location + Width  bit1=0  base1=MSB of Input  bit0=0  base0=LSB of Input  dbl_ovrd=off  block_type=slice
  Slice Enc s2 : xbsIndex_r4/Slice  nbits=1  boolean_output=on  mode=Lower Bit Location + Width  bit1=0  base1=MSB of Input  bit0=3  base0=LSB of Input  dbl_ovrd=off  block_type=slice
  Slice Enc t1 : xbsIndex_r4/Slice  nbits=2  boolean_output=off  mode=Upper Bit Location + Width  bit1=0  base1=MSB of Input  bit0=0  base0=MSB of Input  dbl_ovrd=off  block_type=slice
  Slice Enc t2 : xbsIndex_r4/Slice  nbits=2  boolean_output=off  mode=Lower Bit Location + Width  bit1=0  base1=MSB of Input  bit0=4  base0=LSB of Input  dbl_ovrd=off  block_type=slice
  t1 : Outport
  a1 : Outport  Port=2
  t2 : Outport  Port=3
  a2 : Outport  Port=4
  s2 : Outport  Port=5
  wires:
  Slice Enc t2/1 -> t2/1
  Slice Enc a1/1 -> a1/1
  Slice Enc a2/1 -> a2/1
  Slice Enc t1/1 -> t1/1
  Slice Enc s2/1 -> s2/1
  x/1 -> Slice Enc s2/1, Slice Enc a2/1, Slice Enc t1/1, Slice Enc a1/1, Slice Enc t2/1

== system Karatsuba_Multiplier_64_Unsigned/AE_Multiplier_32_1/Encoder Slicer1 ==
  x : Inport
  Slice Enc a1 : xbsIndex_r4/Slice  nbits=3  boolean_output=off  mode=Lower Bit Location + Width  bit1=0  base1=MSB of Input  bit0=6  base0=LSB of Input  dbl_ovrd=off  block_type=slice
  Slice Enc a2 : xbsIndex_r4/Slice  nbits=3  boolean_output=off  mode=Lower Bit Location + Width  bit1=0  base1=MSB of Input  bit0=0  base0=LSB of Input  dbl_ovrd=off  block_type=slice
  Slice Enc s2 : xbsIndex_r4/Slice  nbits=1  boolean_output=on  mode=Lower Bit Location + Width  bit1=0  base1=MSB of Input  bit0=3  base0=LSB of Input  dbl_ovrd=off  block_type=slice
  Slice Enc t1 : xbsIndex_r4/Slice  nbits=2  boolean_output=off  mode=Upper Bit Location + Width  bit1=0  base1=MSB of Input  bit0=0  base0=MSB of Input  dbl_ovrd=off  block_type=slice
  Slice Enc t2 : xbsIndex_r4/Slice  nbits=2  boolean_output=off  mode=Lower Bit Location + Width  bit1=0  base1=MSB of Input  bit0=4  base0=LSB of Input  dbl_ovrd=off  block_type=slice
  t1 : Outport
  a1 : Outport  Port=2
  t2 : Outport  Port=3
  a2 : Outport  Port=4
  s2 : Outport  Port=5
  wires:
  Slice Enc t2/1 -> t2/1
  Slice Enc a1/1 -> a1/1
  Slice Enc a2/1 -> a2/1
  Slice Enc t1/1 -> t1/1
  Slice Enc s2/1 -> s2/1
  x/1 -> Slice Enc s2/1, Slice Enc a2/1, Slice Enc t1/1, Slice Enc a1/1, Slice Enc t2/1

== system Karatsuba_Multiplier_64_Unsigned/AE_Multiplier_32_1/Encoder Slicer2 ==
  x : Inport
  Slice Enc a1 : xbsIndex_r4/Slice  nbits=3  boolean_output=off  mode=Lower Bit Location + Width  bit1=0  base1=MSB of Input  bit0=6  base0=LSB of Input  dbl_ovrd=off  block_type=slice
  Slice Enc a2 : xbsIndex_r4/Slice  nbits=3  boolean_output=off  mode=Lower Bit Location + Width  bit1=0  base1=MSB of Input  bit0=0  base0=LSB of Input  dbl_ovrd=off  block_type=slice
  Slice Enc s2 : xbsIndex_r4/Slice  nbits=1  boolean_output=on  mode=Lower Bit Location + Width  bit1=0  base1=MSB of Input  bit0=3  base0=LSB of Input  dbl_ovrd=off  block_type=slice
  Slice Enc t1 : xbsIndex_r4/Slice  nbits=2  boolean_output=off  mode=Upper Bit Location + Width  bit1=0  base1=MSB of Input  bit0=0  base0=MSB of Input  dbl_ovrd=off  block_type=slice
  Slice Enc t2 : xbsIndex_r4/Slice  nbits=2  boolean_output=off  mode=Lower Bit Location + Width  bit1=0  base1=MSB of Input  bit0=4  base0=LSB of Input  dbl_ovrd=off  block_type=slice
  t1 : Outport
  a1 : Outport  Port=2
  t2 : Outport  Port=3
  a2 : Outport  Port=4
  s2 : Outport  Port=5
  wires:
  Slice Enc t2/1 -> t2/1
  Slice Enc a1/1 -> a1/1
  Slice Enc a2/1 -> a2/1
  Slice Enc t1/1 -> t1/1
  Slice Enc s2/1 -> s2/1
  x/1 -> Slice Enc s2/1, Slice Enc a2/1, Slice Enc t1/1, Slice Enc a1/1, Slice Enc t2/1

== system Karatsuba_Multiplier_64_Unsigned/AE_Multiplier_32_1/Encoder Slicer3 ==
  x : Inport
  Slice Enc a1 : xbsIndex_r4/Slice  nbits=3  boolean_output=off  mode=Lower Bit Location + Width  bit1=0  base1=MSB of Input  bit0=6  base0=LSB of Input  dbl_ovrd=off  block_type=slice
  Slice Enc a2 : xbsIndex_r4/Slice  nbits=3  boolean_output=off  mode=Lower Bit Location + Width  bit1=0  base1=MSB of Input  bit0=0  base0=LSB of Input  dbl_ovrd=off  block_type=slice
  Slice Enc s2 : xbsIndex_r4/Slice  nbits=1  boolean_output=on  mode=Lower Bit Location + Width  bit1=0  base1=MSB of Input  bit0=3  base0=LSB of Input  dbl_ovrd=off  block_type=slice
  Slice Enc t1 : xbsIndex_r4/Slice  nbits=2  boolean_output=off  mode=Upper Bit Location + Width  bit1=0  base1=MSB of Input  bit0=0  base0=MSB of Input  dbl_ovrd=off  block_type=slice
  Slice Enc t2 : xbsIndex_r4/Slice  nbits=2  boolean_output=off  mode=Lower Bit Location + Width  bit1=0  base1=MSB of Input  bit0=4  base0=LSB of Input  dbl_ovrd=off  block_type=slice
  t1 : Outport
  a1 : Outport  Port=2
  t2 : Outport  Port=3
  a2 : Outport  Port=4
  s2 : Outport  Port=5
  wires:
  Slice Enc t2/1 -> t2/1
  Slice Enc a1/1 -> a1/1
  Slice Enc a2/1 -> a2/1
  Slice Enc t1/1 -> t1/1
  Slice Enc s2/1 -> s2/1
  x/1 -> Slice Enc s2/1, Slice Enc a2/1, Slice Enc t1/1, Slice Enc a1/1, Slice Enc t2/1

== system Karatsuba_Multiplier_64_Unsigned/AE_Multiplier_32_1/Encoder Slicer4 ==
  x : Inport
  Slice Enc a1 : xbsIndex_r4/Slice  nbits=3  boolean_output=off  mode=Lower Bit Location + Width  bit1=0  base1=MSB of Input  bit0=6  base0=LSB of Input  dbl_ovrd=off  block_type=slice
  Slice Enc a2 : xbsIndex_r4/Slice  nbits=3  boolean_output=off  mode=Lower Bit Location + Width  bit1=0  base1=MSB of Input  bit0=0  base0=LSB of Input  dbl_ovrd=off  block_type=slice
  Slice Enc s2 : xbsIndex_r4/Slice  nbits=1  boolean_output=on  mode=Lower Bit Location + Width  bit1=0  base1=MSB of Input  bit0=3  base0=LSB of Input  dbl_ovrd=off  block_type=slice
  Slice Enc t1 : xbsIndex_r4/Slice  nbits=2  boolean_output=off  mode=Upper Bit Location + Width  bit1=0  base1=MSB of Input  bit0=0  base0=MSB of Input  dbl_ovrd=off  block_type=slice
  Slice Enc t2 : xbsIndex_r4/Slice  nbits=2  boolean_output=off  mode=Lower Bit Location + Width  bit1=0  base1=MSB of Input  bit0=4  base0=LSB of Input  dbl_ovrd=off  block_type=slice
  t1 : Outport
  a1 : Outport  Port=2
  t2 : Outport  Port=3
  a2 : Outport  Port=4
  s2 : Outport  Port=5
  wires:
  Slice Enc t2/1 -> t2/1
  Slice Enc a1/1 -> a1/1
  Slice Enc a2/1 -> a2/1
  Slice Enc t1/1 -> t1/1
  Slice Enc s2/1 -> s2/1
  x/1 -> Slice Enc s2/1, Slice Enc a2/1, Slice Enc t1/1, Slice Enc a1/1, Slice Enc t2/1

== system Karatsuba_Multiplier_64_Unsigned/AE_Multiplier_32_2/3B Multiplier ==
  x : Inport
  AddSub : xbsIndex_r4/AddSub  mode=Addition  use_carryin=off  use_carryout=off  en=off  latency=0  precision=User Defined  arith_type=Unsigned  n_bits=64  bin_pt=0  quantization=Truncate  overflow=Wrap  dbl_ovrd=off  use_behavioral_HDL=off  hw_selection=Fabric  pipelined=on  block_type=addsub
  Shift : xbsIndex_r4/Shift  shift_dir=Left  shift_bits=1  en=off  latency=0  precision=User Defined  arith_type=Unsigned  n_bits=64  bin_pt=0  quantization=Truncate  overflow=Wrap  dbl_ovrd=off  block_type=shift
  y : Outport
  wires:
  x/1 -> Shift/1, AddSub/2
  AddSub/1 -> y/1
  Shift/1 -> AddSub/1

== system Karatsuba_Multiplier_64_Unsigned/AE_Multiplier_32_2/5B Multiplier ==
  x : Inport
  AddSub1 : xbsIndex_r4/AddSub  mode=Addition  use_carryin=off  use_carryout=off  en=off  latency=0  precision=User Defined  arith_type=Unsigned  n_bits=64  bin_pt=0  quantization=Truncate  overflow=Wrap  dbl_ovrd=off  use_behavioral_HDL=off  hw_selection=Fabric  pipelined=on  block_type=addsub
  Shift1 : xbsIndex_r4/Shift  shift_dir=Left  shift_bits=2  en=off  latency=0  precision=User Defined  arith_type=Unsigned  n_bits=64  bin_pt=0  quantization=Truncate  overflow=Wrap  dbl_ovrd=off  block_type=shift
  y : Outport
  wires:
  x/1 -> AddSub1/2, Shift1/1
  Shift1/1 -> AddSub1/1
  AddSub1/1 -> y/1

== system Karatsuba_Multiplier_64_Unsigned/AE_Multiplier_32_2/7B Multiplier ==
  x : Inport
  AddSub2 : xbsIndex_r4/AddSub  mode=Subtraction  use_carryin=off  use_carryout=off  en=off  latency=0  precision=User Defined  arith_type=Unsigned  n_bits=64  bin_pt=0  quantization=Truncate  overflow=Wrap  dbl_ovrd=off  use_behavioral_HDL=off  hw_selection=Fabric  pipelined=on  block_type=addsub
  Shift2 : xbsIndex_r4/Shift  shift_dir=Left  shift_bits=3  en=off  latency=0  precision=User Defined  arith_type=Unsigned  n_bits=64  bin_pt=0  quantization=Truncate  overflow=Wrap  dbl_ovrd=off  block_type=shift
  y : Outport
  wires:
  AddSub2/1 -> y/1
  Shift2/1 -> AddSub2/1
  x/1 -> Shift2/1, AddSub2/2

== system Karatsuba_Multiplier_64_Unsigned/AE_Multiplier_32_2/Barrel Shifter 0 ==
  Sel : Inport
  x : Inport  Port=2
  Mux : xbsIndex_r4/Mux  inputs=8  en=off  latency=0  precision=Full  arith_type=Unsigned  n_bits=17  bin_pt=0  quantization=Truncate  overflow=Wrap  dbl_ovrd=off  block_type=mux
  Shift1 : xbsIndex_r4/Shift  shift_dir=Left  shift_bits=1  en=off  latency=0  precision=User Defined  arith_type=Unsigned  n_bits=64  bin_pt=0  quantization=Truncate  overflow=Wrap  dbl_ovrd=off  block_type=shift
  Shift2 : xbsIndex_r4/Shift  shift_dir=Left  shift_bits=2  en=off  latency=0  precision=User Defined  arith_type=Unsigned  n_bits=64  bin_pt=0  quantization=Truncate  overflow=Wrap  dbl_ovrd=off  block_type=shift
  Shift3 : xbsIndex_r4/Shift  shift_dir=Left  shift_bits=3  en=off  latency=0  precision=User Defined  arith_type="Signed  (2's comp)"  n_bits=64  bin_pt=0  quantization=Truncate  overflow=Wrap  dbl_ovrd=off  block_type=shift
  Shift4 : xbsIndex_r4/Shift  shift_dir=Left  shift_bits=4  en=off  latency=0  precision=User Defined  arith_type=Unsigned  n_bits=64  bin_pt=0  quantization=Truncate  overflow=Wrap  dbl_ovrd=off  block_type=shift
  Shift5 : xbsIndex_r4/Shift  shift_dir=Left  shift_bits=5  en=off  latency=0  precision=User Defined  arith_type=Unsigned  n_bits=43  bin_pt=0  quantization=Truncate  overflow=Wrap  dbl_ovrd=off  block_type=shift
  Shift6 : xbsIndex_r4/Shift  shift_dir=Left  shift_bits=6  en=off  latency=0  precision=User Defined  arith_type=Unsigned  n_bits=64  bin_pt=0  quantization=Truncate  overflow=Wrap  dbl_ovrd=off  block_type=shift
  Shift7 : xbsIndex_r4/Shift  shift_dir=Left  shift_bits=7  en=off  latency=0  precision=User Defined  arith_type=Unsigned  n_bits=64  bin_pt=0  quantization=Truncate  overflow=Wrap  dbl_ovrd=off  block_type=shift
  y : Outport
  wires:
  Mux/1 -> y/1
  Sel/1 -> Mux/1
  x/1 -> Shift1/1, Shift2/1, Shift3/1, Shift4/1, Shift5/1, Shift6/1, Shift7/1, Mux/2
  Shift1/1 -> Mux/3
  Shift2/1 -> Mux/4
  Shift3/1 -> Mux/5
  Shift4/1 -> Mux/6
  Shift5/1 -> Mux/7
  Shift6/1 -> Mux/8
  Shift7/1 -> Mux/9

== system Karatsuba_Multiplier_64_Unsigned/AE_Multiplier_32_2/Barrel Shifter 1 ==
  Sel : Inport
  x : Inport  Port=2
  Mux : xbsIndex_r4/Mux  inputs=8  en=off  latency=0  precision=Full  arith_type=Unsigned  n_bits=17  bin_pt=0  quantization=Truncate  overflow=Wrap  dbl_ovrd=off  block_type=mux
  Shift1 : xbsIndex_r4/Shift  shift_dir=Left  shift_bits=1  en=off  latency=0  precision=User Defined  arith_type=Unsigned  n_bits=64  bin_pt=0  quantization=Truncate  overflow=Wrap  dbl_ovrd=off  block_type=shift
  Shift2 : xbsIndex_r4/Shift  shift_dir=Left  shift_bits=2  en=off  latency=0  precision=User Defined  arith_type=Unsigned  n_bits=64  bin_pt=0  quantization=Truncate  overflow=Wrap  dbl_ovrd=off  block_type=shift
  Shift3 : xbsIndex_r4/Shift  shift_dir=Left  shift_bits=3  en=off  latency=0  precision=User Defined  arith_type="Signed  (2's comp)"  n_bits=64  bin_pt=0  quantization=Truncate  overflow=Wrap  dbl_ovrd=off  block_type=shift
  Shift4 : xbsIndex_r4/Shift  shift_dir=Left  shift_bits=4  en=off  latency=0  precision=User Defined  arith_type=Unsigned  n_bits=64  bin_pt=0  quantization=Truncate  overflow=Wrap  dbl_ovrd=off  block_type=shift
  Shift5 : xbsIndex_r4/Shift  shift_dir=Left  shift_bits=5  en=off  latency=0  precision=User Defined  arith_type=Unsigned  n_bits=43  bin_pt=0  quantization=Truncate  overflow=Wrap  dbl_ovrd=off  block_type=shift
  Shift6 : xbsIndex_r4/Shift  shift_dir=Left  shift_bits=6  en=off  latency=0  precision=User Defined  arith_type=Unsigned  n_bits=64  bin_pt=0  quantization=Truncate  overflow=Wrap  dbl_ovrd=off  block_type=shift
  Shift7 : xbsIndex_r4/Shift  shift_dir=Left  shift_bits=7  en=off  latency=0  precision=User Defined  arith_type=Unsigned  n_bits=64  bin_pt=0  quantization=Truncate  overflow=Wrap  dbl_ovrd=off  block_type=shift
  y : Outport
  wires:
  Mux/1 -> y/1
  Sel/1 -> Mux/1
  x/1 -> Shift1/1, Shift2/1, Shift3/1, Shift4/1, Shift5/1, Shift6/1, Shift7/1, Mux/2
  Shift1/1 -> Mux/3
  Shift2/1 -> Mux/4
  Shift3/1 -> Mux/5
  Shift4/1 -> Mux/6
  Shift5/1 -> Mux/7
  Shift6/1 -> Mux/8
  Shift7/1 -> Mux/9

== system Karatsuba_Multiplier_64_Unsigned/AE_Multiplier_32_2/Barrel Shifter 2 ==
  Sel : Inport
  x : Inport  Port=2
  Mux : xbsIndex_r4/Mux  inputs=8  en=off  latency=0  precision=Full  arith_type=Unsigned  n_bits=17  bin_pt=0  quantization=Truncate  overflow=Wrap  dbl_ovrd=off  block_type=mux
  Shift1 : xbsIndex_r4/Shift  shift_dir=Left  shift_bits=1  en=off  latency=0  precision=User Defined  arith_type=Unsigned  n_bits=64  bin_pt=0  quantization=Truncate  overflow=Wrap  dbl_ovrd=off  block_type=shift
  Shift2 : xbsIndex_r4/Shift  shift_dir=Left  shift_bits=2  en=off  latency=0  precision=User Defined  arith_type=Unsigned  n_bits=64  bin_pt=0  quantization=Truncate  overflow=Wrap  dbl_ovrd=off  block_type=shift
  Shift3 : xbsIndex_r4/Shift  shift_dir=Left  shift_bits=3  en=off  latency=0  precision=User Defined  arith_type="Signed  (2's comp)"  n_bits=64  bin_pt=0  quantization=Truncate  overflow=Wrap  dbl_ovrd=off  block_type=shift
  Shift4 : xbsIndex_r4/Shift  shift_dir=Left  shift_bits=4  en=off  latency=0  precision=User Defined  arith_type=Unsigned  n_bits=64  bin_pt=0  quantization=Truncate  overflow=Wrap  dbl_ovrd=off  block_type=shift
  Shift5 : xbsIndex_r4/Shift  shift_dir=Left  shift_bits=5  en=off  latency=0  precision=User Defined  arith_type=Unsigned  n_bits=43  bin_pt=0  quantization=Truncate  overflow=Wrap  dbl_ovrd=off  block_type=shift
  Shift6 : xbsIndex_r4/Shift  shift_dir=Left  shift_bits=6  en=off  latency=0  precision=User Defined  arith_type=Unsigned  n_bits=64  bin_pt=0  quantization=Truncate  overflow=Wrap  dbl_ovrd=off  block_type=shift
  Shift7 : xbsIndex_r4/Shift  shift_dir=Left  shift_bits=7  en=off  latency=0  precision=User Defined  arith_type=Unsigned  n_bits=64  bin_pt=0  quantization=Truncate  overflow=Wrap  dbl_ovrd=off  block_type=shift
  y : Outport
  wires:
  Mux/1 -> y/1
  Sel/1 -> Mux/1
  x/1 -> Shift1/1, Shift2/1, Shift3/1, Shift4/1, Shift5/1, Shift6/1, Shift7/1, Mux/2
  Shift1/1 -> Mux/3
  Shift2/1 -> Mux/4
  Shift3/1 -> Mux/5
  Shift4/1 -> Mux/6
  Shift5/1 -> Mux/7
  Shift6/1 -> Mux/8
  Shift7/1 -> Mux/9

== system Karatsuba_Multiplier_64_Unsigned/AE_Multiplier_32_2/Barrel Shifter 3 ==
  Sel : Inport
  x : Inport  Port=2
  Mux : xbsIndex_r4/Mux  inputs=8  en=off  latency=0  precision=Full  arith_type=Unsigned  n_bits=17  bin_pt=0  quantization=Truncate  overflow=Wrap  dbl_ovrd=off  block_type=mux
  Shift1 : xbsIndex_r4/Shift  shift_dir=Left  shift_bits=1  en=off  latency=0  precision=User Defined  arith_type=Unsigned  n_bits=64  bin_pt=0  quantization=Truncate  overflow=Wrap  dbl_ovrd=off  block_type=shift
  Shift2 : xbsIndex_r4/Shift  shift_dir=Left  shift_bits=2  en=off  latency=0  precision=User Defined  arith_type=Unsigned  n_bits=64  bin_pt=0  quantization=Truncate  overflow=Wrap  dbl_ovrd=off  block_type=shift
  Shift3 : xbsIndex_r4/Shift  shift_dir=Left  shift_bits=3  en=off  latency=0  precision=User Defined  arith_type="Signed  (2's comp)"  n_bits=64  bin_pt=0  quantization=Truncate  overflow=Wrap  dbl_ovrd=off  block_type=shift
  Shift4 : xbsIndex_r4/Shift  shift_dir=Left  shift_bits=4  en=off  latency=0  precision=User Defined  arith_type=Unsigned  n_bits=64  bin_pt=0  quantization=Truncate  overflow=Wrap  dbl_ovrd=off  block_type=shift
  Shift5 : xbsIndex_r4/Shift  shift_dir=Left  shift_bits=5  en=off  latency=0  precision=User Defined  arith_type=Unsigned  n_bits=43  bin_pt=0  quantization=Truncate  overflow=Wrap  dbl_ovrd=off  block_type=shift
  Shift6 : xbsIndex_r4/Shift  shift_dir=Left  shift_bits=6  en=off  latency=0  precision=User Defined  arith_type=Unsigned  n_bits=64  bin_pt=0  quantization=Truncate  overflow=Wrap  dbl_ovrd=off  block_type=shift
  Shift7 : xbsIndex_r4/Shift  shift_dir=Left  shift_bits=7  en=off  latency=0  precision=User Defined  arith_type=Unsigned  n_bits=64  bin_pt=0  quantization=Truncate  overflow=Wrap  dbl_ovrd=off  block_type=shift
  y : Outport
  wires:
  Mux/1 -> y/1
  Sel/1 -> Mux/1
  x/1 -> Shift1/1, Shift2/1, Shift3/1, Shift4/1, Shift5/1, Shift6/1, Shift7/1, Mux/2
  Shift1/1 -> Mux/3
  Shift2/1 -> Mux/4
  Shift3/1 -> Mux/5
  Shift4/1 -> Mux/6
  Shift5/1 -> Mux/7
  Shift6/1 -> Mux/8
  Shift7/1 -> Mux/9
